simulink model "ArduCopter_MinnieDieterController"  (R2018b)
settings: Solver=FixedStepDiscrete  StartTime=0.0  StopTime=1000  FixedStep=cntrl.sample_time  RelTol=1e-4
libraries: ardupilot_custom_controller_lib x2, axes_transformation_lib x2, simulink x1, fmCopterDieterIndi_lib x1
settings Model: DataTypeOverride=Single  DataTypeOverrideAppliesTo=Floating-point  Creator=Yannic  LastModifiedBy=eike
settings SolverCC: ZeroCrossControl=DisableAll
settings DataIOCC: LimitDataPoints=on  SaveOutput=off  SaveTime=off  ReturnWorkspaceOutputs=on
settings OptimizationCC: DefaultParameterBehavior=Inlined  UseFloatMulNetSlope=on  DefaultUnderspecifiedDataType=single  InlineInvariantSignals=on  PassReuseOutputArgsAs=Individual arguments  ZeroExternalMemoryAtStartup=off  ZeroInternalMemoryAtStartup=off  NoFixptDivByZeroProtection=on  EfficientFloat2IntCast=on  LifeSpan=1  OptimizeBlockOrder=speed  DifferentSizesBufferReuse=on
settings DebuggingCC: ReadBeforeWriteMsg=DisableAll  WriteAfterWriteMsg=DisableAll  WriteAfterReadMsg=DisableAll  MultiTaskDSMMsg=none  ParameterPrecisionLossMsg=none  ParameterTunabilityLossMsg=error  AllowSymbolicDim=off  LibraryContextMissingDiagnostic=none  SFUnexpectedBacktrackingDiag=warning  SFNoUnconditionalDefaultTransitionDiag=warning  SFExecutionAtInitializationDiag=none  UnderSpecifiedDimensionMsg=warning
settings HardwareCC: ProdBitPerPointer=32  ProdBitPerSizeT=32  ProdBitPerPtrDiffT=32  ProdLargestAtomicInteger=Long  ProdWordSize=32  ProdHWDeviceType=ARM Compatible->ARM 7
settings ModelReferenceCC: UpdateModelReferenceTargets=IfOutOfDate  PropagateSignalLabelsOutOfModel=off
settings SFSimCC: SFSimEcho=off  SimUseLocalCustomCode=off  MATLABDynamicMemAlloc=off
settings RTWCC: SystemTargetFile=ert.tlc  GenCodeOnly=on  TemplateMakefile=ert_default_tmf  GenerateReport=on  RTWUseLocalCustomCode=off  IncludeHyperlinkInReport=on  LaunchReport=on  TargetLang=C++  GenerateTraceInfo=on  GenerateTraceReport=on  GenerateTraceReportSl=on  GenerateTraceReportSf=on  GenerateTraceReportEml=on
settings CodeAppCC: ForceParamTrailComments=on  IgnoreCustomStorageClasses=off  OperatorAnnotations=on  SimulinkDataObjDesc=on  SFDataObjDesc=on  CustomSymbolStrGlobalVar=rt$N$M  CustomSymbolStrType=$N$M  CustomSymbolStrFcn=$N$M$F  CustomSymbolStrMacro=$N$M  InsertBlockDesc=on
settings ERTTargetCC: TargetLangStandard=C++03 (ISO)  GenerateSampleERTMain=on  IncludeMdlTerminateFcn=off  CombineSignalStateStructs=on  SuppressErrorStatus=on  SupportAbsoluteTime=off  MultiInstanceERTCode=on  CodeInterfacePackaging=C++ class  SupportVariableSizeSignals=on  ERTHeaderFileRootName=MatlabController$E  ERTSourceFileRootName=MatlabController$E  ERTDataFileRootName=MatlabController_data  InlinedParameterPlacement=NonHierarchical  RootIOFormat=Structure reference  ERTCustomFileTemplate=example_file_process.tlc  ERTFilePackagingFormat=CompactWithDataFile
settings ConfigComp: CovMetricSettings=dw  CovHtmlReporting=on  CovSaveCumulativeToWorkspaceVar=on  CovSaveSingleToWorkspaceVar=on  CovExternalEMLEnable=off

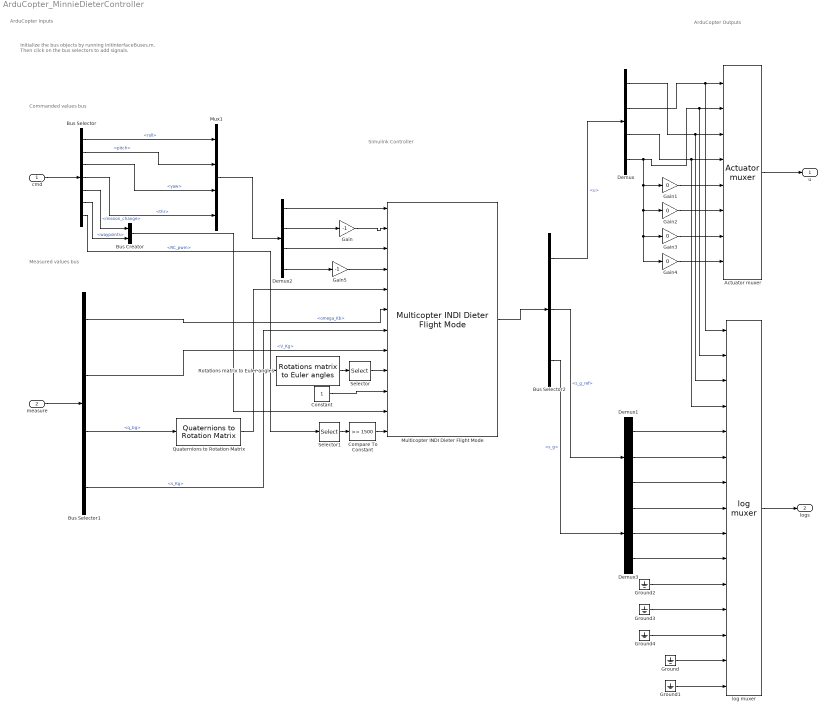
== system ArduCopter_MinnieDieterController ==
  note: Measured values bus
  note: Initialize the bus objects by running initInterfaceBuses.m.
      | Then click on the bus selectors to add signals.
  note: Commanded values bus
  note: ArduCopter Inputs
  note: ArduCopter Outputs
  note: Simulink Controller
  cmd : Inport  OutDataTypeStr=Bus: cmdBus
  measure : Inport  Port=2  OutDataTypeStr=Bus: measureBus
  Actuator muxer : ardupilot_custom_controller_lib/Actuator muxer
      settings: SourceProductName=LADAC
  Bus Creator : BusCreator  Inputs=2
  Bus Selector : BusSelector  OutputSignals=roll,pitch,yaw,thr,mission_change,waypoints,RC_pwm
  Bus Selector1 : BusSelector  OutputSignals=omega_Kb,V_Kg,q_bg,s_Kg
  Bus Selector2 : BusSelector  OutputSignals=u,pos_cntrl.reference.s_g_ref,pos_cntrl.measure.s_g
  Compare To Constant : simulink/Logic and Bit Operations/Compare To Constant  relop=>=  const=1500  OutDataTypeStr=uint8
  Constant : Constant
  Demux : Demux
  Demux1 : Demux  Outputs=3
  Demux2 : Demux
  Demux3 : Demux  Outputs=3
  Gain : Gain  Gain=-1
  Gain{1..4} (4 alike) : Gain  Gain=0
  Gain5 : Gain  Gain=-1
  Ground{,1..4} (5 alike) : Ground
  Multicopter INDI Dieter Flight Mode : fmCopterDieterIndi_lib/Multicopter INDI Dieter Flight Mode  fm=fm_Traj
  Mux1 : Mux
  Quaternions to Rotation Matrix : axes_transformation_lib/Quaternions to Rotation Matrix  SystemSampleTime=-1
      settings: SourceProductName=LADAC
  Rotations matrix to Euler angles : axes_transformation_lib/Rotations matrix to Euler angles  SystemSampleTime=-1
      settings: SourceProductName=LADAC
  Selector : Selector  InputPortWidth=3  IndexOptions=Index vector (dialog)  Indices=3  OutputSizes=1
  Selector1 : Selector  InputPortWidth=16  IndexOptions=Index vector (dialog)  Indices=7  OutputSizes=1
  log muxer : ardupilot_custom_controller_lib/log muxer
      settings: SourceProductName=LADAC
  u : Outport
  logs : Outport  Port=2
  wires:
  cmd/1 -> Bus Selector/1
  measure/1 -> Bus Selector1/1
  Bus Selector/1 -> Mux1/1  "<roll>"
  Bus Selector/2 -> Mux1/2  "<pitch>"
  Bus Selector/3 -> Mux1/3  "<yaw>"
  Bus Selector/4 -> Mux1/4  "<thr>"
  Actuator muxer/1 -> u/1
  log muxer/1 -> logs/1
  Gain1/1 -> Actuator muxer/5
  Demux/2 -> log muxer/1, Actuator muxer/1
  Demux/4 -> log muxer/2, Actuator muxer/2, Gain1/1, Gain4/1, Gain3/1, Gain2/1
  Demux/1 -> log muxer/3, Actuator muxer/3
  Demux/3 -> log muxer/4, Actuator muxer/4
  Demux1/1 -> log muxer/5
  Demux1/2 -> log muxer/6
  Demux1/3 -> log muxer/7
  Demux3/1 -> log muxer/8
  Demux3/2 -> log muxer/9
  Demux3/3 -> log muxer/10
  Ground2/1 -> log muxer/11
  Ground3/1 -> log muxer/12
  Ground4/1 -> log muxer/13
  Ground/1 -> log muxer/14
  Ground1/1 -> log muxer/15
  Gain/1 -> Multicopter INDI Dieter Flight Mode/2
  Quaternions to Rotation Matrix/1 -> Multicopter INDI Dieter Flight Mode/5, Rotations matrix to Euler angles/1
  Bus Selector1/2 -> Multicopter INDI Dieter Flight Mode/8  "<V_Kg>"
  Demux2/4 -> Gain5/1
  Rotations matrix to Euler angles/1 -> Selector/1
  Mux1/1 -> Demux2/1
  Bus Selector1/1 -> Multicopter INDI Dieter Flight Mode/6  "<omega_Kb>"
  Demux2/2 -> Gain/1
  Demux2/3 -> Multicopter INDI Dieter Flight Mode/3
  Bus Selector1/4 -> Multicopter INDI Dieter Flight Mode/7  "<s_Kg>"
  Constant/1 -> Multicopter INDI Dieter Flight Mode/10
  Demux2/1 -> Multicopter INDI Dieter Flight Mode/1
  Bus Selector1/3 -> Quaternions to Rotation Matrix/1  "<q_bg>"
  Multicopter INDI Dieter Flight Mode/1 -> Bus Selector2/1
  Bus Selector2/1 -> Demux/1  "<u>"
  Gain2/1 -> Actuator muxer/6
  Gain3/1 -> Actuator muxer/7
  Gain4/1 -> Actuator muxer/8
  Selector/1 -> Multicopter INDI Dieter Flight Mode/9
  Bus Selector/5 -> Bus Creator/1  "<mission_change>"
  Bus Selector/6 -> Bus Creator/2  "<waypoints>"
  Bus Creator/1 -> Multicopter INDI Dieter Flight Mode/11
  Bus Selector/7 -> Selector1/1  "<RC_pwm>"
  Compare To Constant/1 -> Multicopter INDI Dieter Flight Mode/12
  Selector1/1 -> Compare To Constant/1
  Bus Selector2/2 -> Demux1/1  "<s_g_ref>"
  Bus Selector2/3 -> Demux3/1  "<s_g>"
  Gain5/1 -> Multicopter INDI Dieter Flight Mode/4
